simulink model "HydraulicSystem"  (R2020a)
settings: Solver=VariableStepAuto  StartTime=0.0  StopTime=10.0  RelTol=1e-3
values from neighbouring files (symbols this model uses):
  A = [ ... (first row only)    [P1_3.m]    (also in P1_4.m = 10)
  g = 9.81    [P2_1.m]
undefined symbols (not defined in the file or in its folder): h_0, R_l, R_r, rho, sgn
settings Model: Creator=Minghong.Xu19  LastModifiedBy=Minghong.Xu19

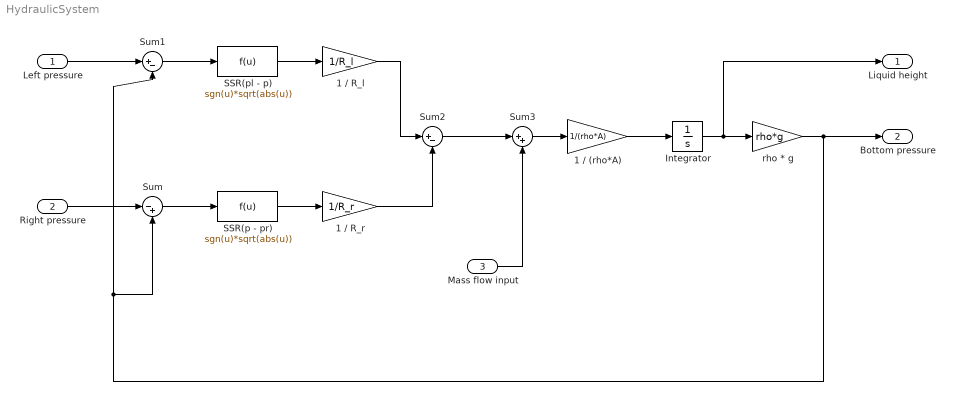
== system HydraulicSystem ==
  Left pressure : Inport
  Right pressure : Inport  Port=2
  Mass flow input : Inport  Port=3
  1 / (rho*A) : Gain  Gain=1/(rho*A)
  1 / R_l : Gain  Gain=1/R_l
  1 / R_r : Gain  Gain=1/R_r
  Integrator : Integrator  InitialCondition=h_0
  SSR(p - pr) : Fcn  Expr=sgn(u)*sqrt(abs(u))
  SSR(pl - p) : Fcn  Expr=sgn(u)*sqrt(abs(u))
  Sum : Sum  Inputs=|-+
  Sum1 : Sum  Inputs=|+-
  Sum2 : Sum  Inputs=|+-
  Sum3 : Sum  Inputs=|++
  rho * g : Gain  Gain=rho*g
  Liquid height : Outport
  Bottom pressure : Outport  Port=2
  wires:
  1 / R_r/1 -> Sum2/2
  rho * g/1 -> Sum/2, Sum1/2, Bottom pressure/1
  Left pressure/1 -> Sum1/1
  1 / (rho*A)/1 -> Integrator/1
  Mass flow input/1 -> Sum3/2
  Sum3/1 -> 1 / (rho*A)/1
  SSR(pl - p)/1 -> 1 / R_l/1
  Right pressure/1 -> Sum/1
  1 / R_l/1 -> Sum2/1
  SSR(p - pr)/1 -> 1 / R_r/1
  Integrator/1 -> rho * g/1, Liquid height/1
  Sum/1 -> SSR(p - pr)/1
  Sum1/1 -> SSR(pl - p)/1
  Sum2/1 -> Sum3/1
